simulink model "c_code_MR100"  (R2023a)
settings: Solver=VariableStepDiscrete  StartTime=0.0  StopTime=inf  MaxStep=0.001  RelTol=1e-3
(part 1 of 4)
settings Model: Creator=LJL  LastModifiedBy=LJL
settings OptimizationCC: DefaultParameterBehavior=Inlined  EnhancedBackFolding=on  PassReuseOutputArgsAs=Individual arguments  ZeroExternalMemoryAtStartup=off  ZeroInternalMemoryAtStartup=off  OptimizeBlockOrder=speed  DifferentSizesBufferReuse=on  OptimizationCustomize=off  EfficientTunableParamExpr=on
settings DebuggingCC: ParameterTunabilityLossMsg=error
settings SFSimCC: MATLABDynamicMemAlloc=off
settings RTWCC: Description=Embedded Coder  SystemTargetFile=ert.tlc  PackageGeneratedCodeAndArtifacts=on  TemplateMakefile=ert_default_tmf  GenerateReport=on  LaunchReport=on
settings CodeAppCC: ForceParamTrailComments=on  IgnoreCustomStorageClasses=off  OperatorAnnotations=on  SimulinkDataObjDesc=on  SFDataObjDesc=on  InsertBlockDesc=on
settings ERTTargetCC: TargetLangStandard=C99 (ISO)  GenerateSampleERTMain=on  InlinedParameterPlacement=NonHierarchical  ERTCustomFileTemplate=example_file_process.tlc

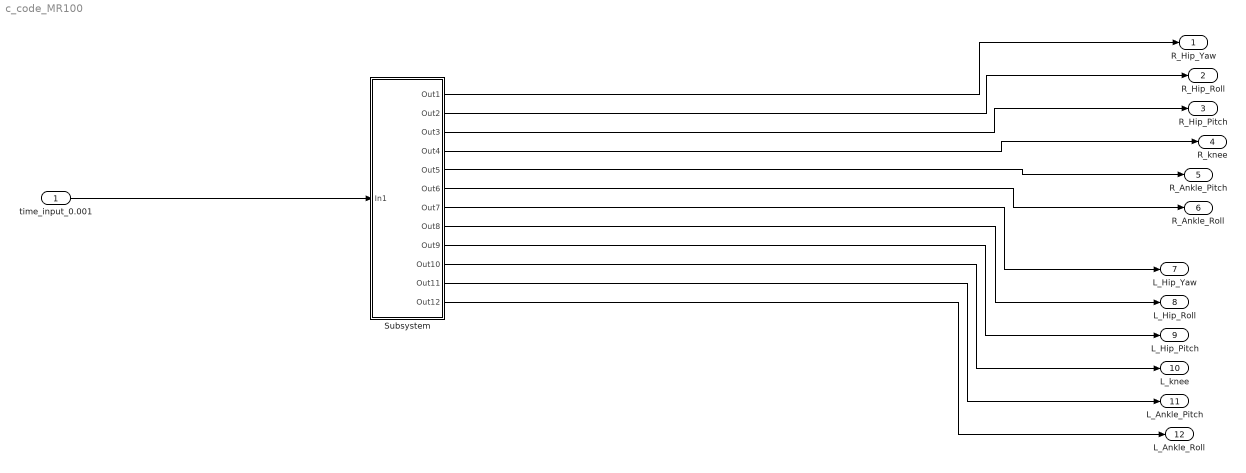
== system c_code_MR100 ==
  time_input_0.001 : Inport
  Subsystem : Subsystem
  R_Hip_Yaw : Outport
  R_Hip_Roll : Outport  Port=2
  R_Hip_Pitch : Outport  Port=3
  R_knee : Outport  Port=4
  R_Ankle_Pitch : Outport  Port=5
  R_Ankle_Roll : Outport  Port=6
  L_Hip_Yaw : Outport  Port=7
  L_Hip_Roll : Outport  Port=8
  L_Hip_Pitch : Outport  Port=9
  L_knee : Outport  Port=10
  L_Ankle_Pitch : Outport  Port=11
  L_Ankle_Roll : Outport  Port=12
  wires:
  time_input_0.001/1 -> Subsystem/1(In1)
  Subsystem/1(Out1) -> R_Hip_Yaw/1
  Subsystem/2(Out2) -> R_Hip_Roll/1
  Subsystem/3(Out3) -> R_Hip_Pitch/1
  Subsystem/4(Out4) -> R_knee/1
  Subsystem/5(Out5) -> R_Ankle_Pitch/1
  Subsystem/6(Out6) -> R_Ankle_Roll/1
  Subsystem/7(Out7) -> L_Hip_Yaw/1
  Subsystem/8(Out8) -> L_Hip_Roll/1
  Subsystem/9(Out9) -> L_Hip_Pitch/1
  Subsystem/10(Out10) -> L_knee/1
  Subsystem/11(Out11) -> L_Ankle_Pitch/1
  Subsystem/12(Out12) -> L_Ankle_Roll/1

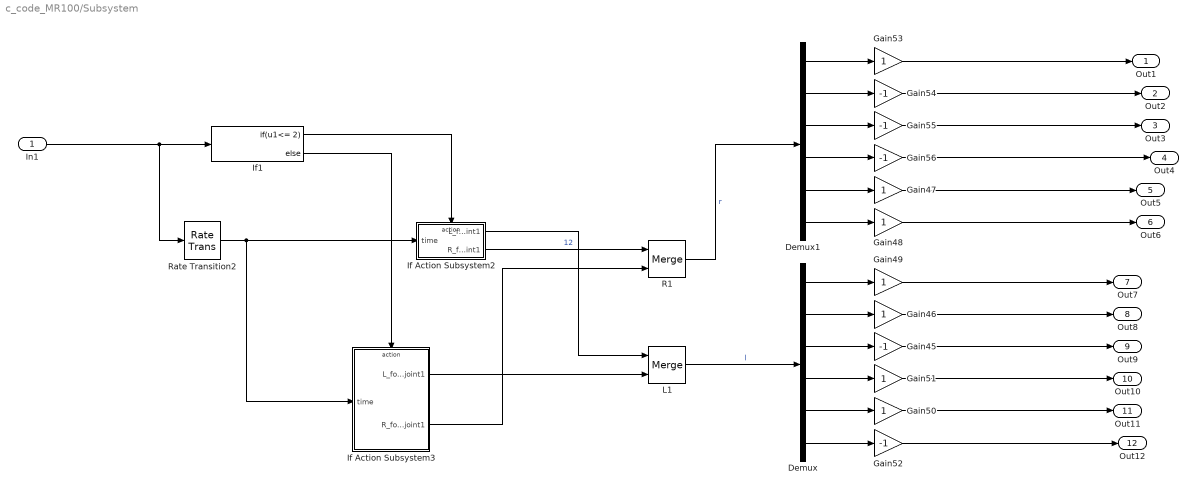
== system c_code_MR100/Subsystem ==
  In1 : Inport
  Demux : Demux  Outputs=6
  Demux1 : Demux  Outputs=6
  Gain{45,52,54..56} (5 alike) : Gain  Gain=-1
  Gain{46..51,53} (7 alike) : Gain
  If Action Subsystem2 : Subsystem  TreatAsAtomicUnit=on
  If Action Subsystem3 : Subsystem  TreatAsAtomicUnit=on
  If1 : If  IfExpression=u1<= 2
  L1 : Merge
  R1 : Merge
  Rate Transition2 : RateTransition  OutPortSampleTime=0.01
  Out1 : Outport
  Out2 : Outport  Port=2
  Out3 : Outport  Port=3
  Out4 : Outport  Port=4
  Out5 : Outport  Port=5
  Out6 : Outport  Port=6
  Out7 : Outport  Port=7
  Out8 : Outport  Port=8
  Out9 : Outport  Port=9
  Out10 : Outport  Port=10
  Out11 : Outport  Port=11
  Out12 : Outport  Port=12
  wires:
  Demux/1 -> Gain49/1
  Demux1/2 -> Gain54/1
  If Action Subsystem2/2(R_foot_joint1) -> R1/1  "12"
  Gain52/1 -> Out12/1
  Demux/4 -> Gain51/1
  Demux/6 -> Gain52/1
  Demux/5 -> Gain50/1
  In1/1 -> Rate Transition2/1, If1/1
  If Action Subsystem3/2(R_foot_joint1) -> R1/2
  Rate Transition2/1 -> If Action Subsystem3/1(time), If Action Subsystem2/1(time)
  Demux/2 -> Gain46/1
  If Action Subsystem2/1(L_foot_joint1) -> L1/1
  Demux/3 -> Gain45/1
  Gain46/1 -> Out8/1
  Demux1/3 -> Gain55/1
  Demux1/4 -> Gain56/1
  L1/1 -> Demux/1  "l"
  If1/1 -> If Action Subsystem2/Action
  Demux1/1 -> Gain53/1
  Gain50/1 -> Out11/1
  Demux1/5 -> Gain47/1
  Gain48/1 -> Out6/1
  Demux1/6 -> Gain48/1
  R1/1 -> Demux1/1  "r"
  Gain55/1 -> Out3/1
  If1/2 -> If Action Subsystem3/Action
  Gain54/1 -> Out2/1
  If Action Subsystem3/1(L_foot_joint1) -> L1/2
  Gain56/1 -> Out4/1
  Gain51/1 -> Out10/1
  Gain53/1 -> Out1/1
  Gain47/1 -> Out5/1
  Gain49/1 -> Out7/1
  Gain45/1 -> Out9/1
